simulink model "wsch_task"  (Simulink 3.00)
libraries: paramlib x357, logiclib x64, mathlib x53, execlib x22, genlib x3, analoglib x3

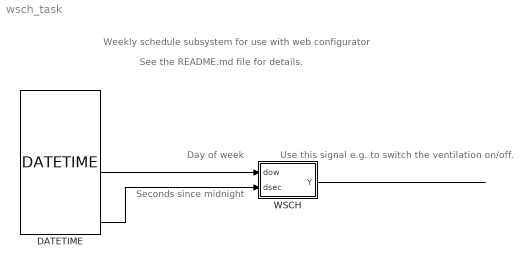
== system wsch_task ==
  note: Weekly schedule subsystem for use with web configurator
  note: See the README.md file for details.
  note: Day of week
  note: Seconds since midnight
  note: Use this signal e.g. to
      | switch the ventilation on/off.
  DATETIME : execlib/DATETIME  isetmode=1: OS clock  igetmode=1: OS clock  settol=1  setper=0  getper=1  FDOW=off  tz=1: Local time
  WSCH : Subsystem
      mask Type: REX sequence
  wires:
  DATETIME/8 -> WSCH/1(dow)
  DATETIME/13 -> WSCH/2(dsec)
  WSCH/1(Y) -> ?

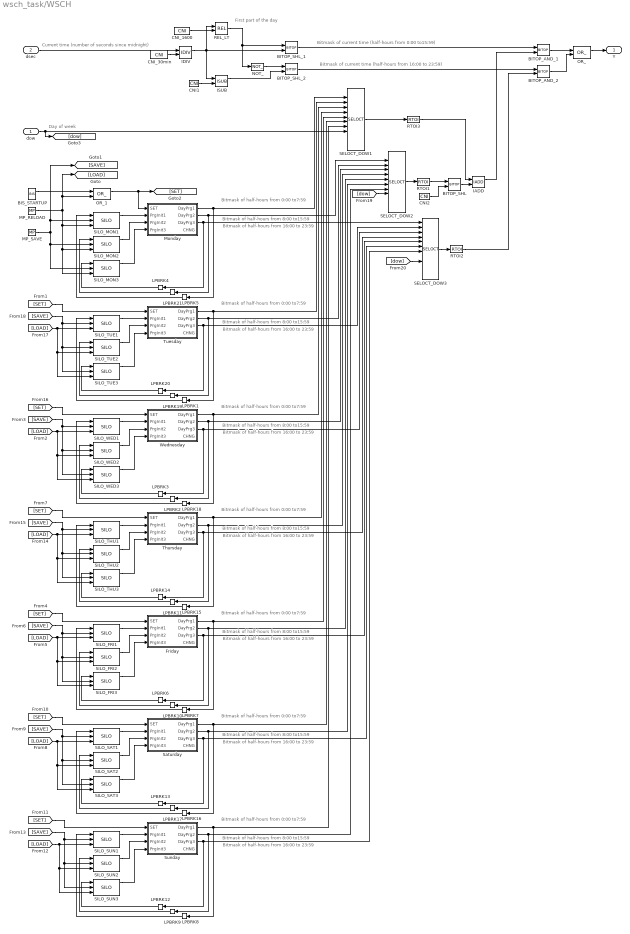
== system wsch_task/WSCH ==
  note: Bitmask of current time (half-hours from 0:00 to15:59)
  note: Bitmask of current time (half-hours from 16:00 to 23:59)
  note: First part of the day
  note: Bitmask of half-hours from 16:00 to 23:59
  note: Current time (number of seconds since midnight)
  note: Day of week
  note: Bitmask of half-hours from 0:00 to7:59
  note: Bitmask of half-hours from 8:00 to15:59
  note: Bitmask of half-hours from 16:00 to 23:59
  note: Bitmask of half-hours from 0:00 to7:59
  note: Bitmask of half-hours from 8:00 to15:59
  note: Bitmask of half-hours from 16:00 to 23:59
  note: Bitmask of half-hours from 0:00 to7:59
  note: Bitmask of half-hours from 8:00 to15:59
  note: Bitmask of half-hours from 16:00 to 23:59
  note: Bitmask of half-hours from 0:00 to7:59
  note: Bitmask of half-hours from 8:00 to15:59
  note: Bitmask of half-hours from 16:00 to 23:59
  note: Bitmask of half-hours from 0:00 to7:59
  note: Bitmask of half-hours from 8:00 to15:59
  note: Bitmask of half-hours from 16:00 to 23:59
  note: Bitmask of half-hours from 0:00 to7:59
  note: Bitmask of half-hours from 8:00 to15:59
  note: Bitmask of half-hours from 16:00 to 23:59
  note: Bitmask of half-hours from 0:00 to7:59
  note: Bitmask of half-hours from 8:00 to15:59
  dow : Inport  Port=1
  dsec : Inport  Port=2
  BIS_STARTUP : genlib/BIS  Y0=off  t1=1  t2=2  t3=0  t4=4  t5=5  t6=6  t7=7  t8=8  RPT=off
  BITOP_AND_1 : logiclib/BITOP  iop=3: Bit AND
  BITOP_AND_2 : logiclib/BITOP  iop=3: Bit AND
  BITOP_SHL : logiclib/BITOP  iop=5: Shift Left
  BITOP_SHL_1 : logiclib/BITOP  iop=5: Shift Left
  BITOP_SHL_2 : logiclib/BITOP  iop=5: Shift Left
  CNI1 : mathlib/CNI  icn=32
  CNI2 : mathlib/CNI  icn=16
  CNI_1600 : mathlib/CNI  icn=32
  CNI_30min : mathlib/CNI  icn=1800
  Friday : Subsystem
      mask Type: REX sequence
  IADD : mathlib/IADD  vtype=4: Long  SAT=off
  IDIV : mathlib/IDIV  vtype=4: Long  nerr=1
  ISUB : mathlib/ISUB  vtype=4: Long  SAT=off
  LPBRK{1..21} (21 alike) : execlib/LPBRK  Orientation=left
  MP_RELOAD : genlib/MP  pwidth=1  BSTATE=off  RPTF=off
  MP_SAVE : genlib/MP  pwidth=1  BSTATE=off  RPTF=off
  Monday : Subsystem
      mask Type: REX sequence
  NOT_ : logiclib/NOT_
  OR_ : logiclib/OR_
  OR_1 : logiclib/OR_
  REL_LT : mathlib/REL  irel=3: less than (<)
  RTOI1 : mathlib/RTOI
  RTOI2 : mathlib/RTOI
  RTOI3 : mathlib/RTOI
  SELOCT_DOW1 : analoglib/SELOCT  BINF=off
  SELOCT_DOW2 : analoglib/SELOCT  BINF=off
  SELOCT_DOW3 : analoglib/SELOCT  BINF=off
  SILO_FRI1 : paramlib/SILO  fname=wschfilt_fri1.dat  CSF=off  CLF=off  yerr=0
  SILO_FRI2 : paramlib/SILO  fname=wschfilt_fri2.dat  CSF=off  CLF=off  yerr=0
  SILO_FRI3 : paramlib/SILO  fname=wschfilt_fri3.dat  CSF=off  CLF=off  yerr=0
  SILO_MON1 : paramlib/SILO  fname=wschfilt_mon1.dat  CSF=off  CLF=off  yerr=0
  SILO_MON2 : paramlib/SILO  fname=wschfilt_mon2.dat  CSF=off  CLF=off  yerr=0
  SILO_MON3 : paramlib/SILO  fname=wschfilt_mon3.dat  CSF=off  CLF=off  yerr=0
  SILO_SAT1 : paramlib/SILO  fname=wschfilt_sat1.dat  CSF=off  CLF=off  yerr=0
  SILO_SAT2 : paramlib/SILO  fname=wschfilt_sat2.dat  CSF=off  CLF=off  yerr=0
  SILO_SAT3 : paramlib/SILO  fname=wschfilt_sat3.dat  CSF=off  CLF=off  yerr=0
  SILO_SUN1 : paramlib/SILO  fname=wschfilt_sun1.dat  CSF=off  CLF=off  yerr=0
  SILO_SUN2 : paramlib/SILO  fname=wschfilt_sun2.dat  CSF=off  CLF=off  yerr=0
  SILO_SUN3 : paramlib/SILO  fname=wschfilt_sun3.dat  CSF=off  CLF=off  yerr=0
  SILO_THU1 : paramlib/SILO  fname=wschfilt_thu1.dat  CSF=off  CLF=off  yerr=0
  SILO_THU2 : paramlib/SILO  fname=wschfilt_thu2.dat  CSF=off  CLF=off  yerr=0
  SILO_THU3 : paramlib/SILO  fname=wschfilt_thu3.dat  CSF=off  CLF=off  yerr=0
  SILO_TUE1 : paramlib/SILO  fname=wschfilt_tue1.dat  CSF=off  CLF=off  yerr=0
  SILO_TUE2 : paramlib/SILO  fname=wschfilt_tue2.dat  CSF=off  CLF=off  yerr=0
  SILO_TUE3 : paramlib/SILO  fname=wschfilt_tue3.dat  CSF=off  CLF=off  yerr=0
  SILO_WED1 : paramlib/SILO  fname=wschfilt_wed1.dat  CSF=off  CLF=off  yerr=0
  SILO_WED2 : paramlib/SILO  fname=wschfilt_wed2.dat  CSF=off  CLF=off  yerr=0
  SILO_WED3 : paramlib/SILO  fname=wschfilt_wed3.dat  CSF=off  CLF=off  yerr=0
  Saturday : Subsystem
      mask Type: REX sequence
  Sunday : Subsystem
      mask Type: REX sequence
  Thursday : Subsystem
      mask Type: REX sequence
  Tuesday : Subsystem
      mask Type: REX sequence
  Wednesday : Subsystem
      mask Type: REX sequence
  Y : Outport  Port=1
  wires:
  BIS_STARTUP/1 -> OR_1/1
  BITOP_AND_1/1 -> OR_/1
  BITOP_AND_2/1 -> OR_/2
  BITOP_SHL/1 -> IADD/2
  BITOP_SHL_1/1 -> BITOP_AND_1/1
  BITOP_SHL_2/1 -> BITOP_AND_2/1
  CNI1/1 -> ISUB/2
  CNI2/1 -> BITOP_SHL/2
  CNI_1600/1 -> REL_LT/2
  CNI_30min/1 -> IDIV/2
  Friday/1(DayPrg1) -> LPBRK7/1, SELOCT_DOW1/6
  Friday/2(DayPrg2) -> LPBRK10/1, SELOCT_DOW2/6
  Friday/3(DayPrg3) -> LPBRK6/1, SELOCT_DOW3/5
  [SET] -> Tuesday/1(SET)
  [SET] -> Saturday/1(SET)
  [SET] -> Sunday/1(SET)
  [LOAD] -> SILO_SUN1/3, SILO_SUN2/3, SILO_SUN3/3
  [SAVE] -> SILO_SUN1/2, SILO_SUN2/2, SILO_SUN3/2
  [LOAD] -> SILO_THU1/3, SILO_THU2/3, SILO_THU3/3
  [SAVE] -> SILO_THU1/2, SILO_THU2/2, SILO_THU3/2
  [SET] -> Wednesday/1(SET)
  [LOAD] -> SILO_TUE1/3, SILO_TUE2/3, SILO_TUE3/3
  [SAVE] -> SILO_TUE1/2, SILO_TUE2/2, SILO_TUE3/2
  [dow] -> SELOCT_DOW2/9
  [LOAD] -> SILO_WED1/3, SILO_WED2/3, SILO_WED3/3
  [dow] -> SELOCT_DOW3/9
  [SAVE] -> SILO_WED1/2, SILO_WED2/2, SILO_WED3/2
  [SET] -> Friday/1(SET)
  [LOAD] -> SILO_FRI1/3, SILO_FRI2/3, SILO_FRI3/3
  [SAVE] -> SILO_FRI1/2, SILO_FRI2/2, SILO_FRI3/2
  [SET] -> Thursday/1(SET)
  [LOAD] -> SILO_SAT1/3, SILO_SAT2/3, SILO_SAT3/3
  [SAVE] -> SILO_SAT1/2, SILO_SAT2/2, SILO_SAT3/2
  IADD/1 -> BITOP_AND_1/2
  IDIV/1 -> BITOP_SHL_1/2, ISUB/1, REL_LT/1
  ISUB/1 -> BITOP_SHL_2/2
  LPBRK1/1 -> SILO_TUE1/1
  LPBRK10/1 -> SILO_FRI2/1
  LPBRK11/1 -> SILO_THU2/1
  LPBRK12/1 -> SILO_SUN3/1
  LPBRK13/1 -> SILO_SAT3/1
  LPBRK14/1 -> SILO_THU3/1
  LPBRK15/1 -> SILO_THU1/1
  LPBRK16/1 -> SILO_SAT1/1
  LPBRK17/1 -> SILO_SAT2/1
  LPBRK18/1 -> SILO_WED1/1
  LPBRK19/1 -> SILO_TUE2/1
  LPBRK2/1 -> SILO_WED2/1
  LPBRK20/1 -> SILO_TUE3/1
  LPBRK21/1 -> SILO_MON2/1
  LPBRK3/1 -> SILO_WED3/1
  LPBRK4/1 -> SILO_MON3/1
  LPBRK5/1 -> SILO_MON1/1
  LPBRK6/1 -> SILO_FRI3/1
  LPBRK7/1 -> SILO_FRI1/1
  LPBRK8/1 -> SILO_SUN1/1
  LPBRK9/1 -> SILO_SUN2/1
  MP_RELOAD/1 -> SILO_MON1/3, SILO_MON2/3, SILO_MON3/3, [LOAD], OR_1/2
  MP_SAVE/1 -> [SAVE], SILO_MON1/2, SILO_MON2/2, SILO_MON3/2
  Monday/1(DayPrg1) -> LPBRK5/1, SELOCT_DOW1/2
  Monday/2(DayPrg2) -> LPBRK21/1, SELOCT_DOW2/2
  Monday/3(DayPrg3) -> LPBRK4/1, SELOCT_DOW3/1
  NOT_/1 -> BITOP_SHL_2/1
  OR_/1 -> Y/1
  OR_1/1 -> [SET], Monday/1(SET)
  REL_LT/1 -> BITOP_SHL_1/1, NOT_/1
  RTOI1/1 -> BITOP_SHL/1
  RTOI2/1 -> BITOP_AND_2/2
  RTOI3/1 -> IADD/1
  SELOCT_DOW1/1 -> RTOI3/1
  SELOCT_DOW2/1 -> RTOI1/1
  SELOCT_DOW3/1 -> RTOI2/1
  SILO_FRI1/1 -> Friday/2(PrgInit1)
  SILO_FRI2/1 -> Friday/3(PrgInit2)
  SILO_FRI3/1 -> Friday/4(PrgInit3)
  SILO_MON1/1 -> Monday/2(PrgInit1)
  SILO_MON2/1 -> Monday/3(PrgInit2)
  SILO_MON3/1 -> Monday/4(PrgInit3)
  SILO_SAT1/1 -> Saturday/2(PrgInit1)
  SILO_SAT2/1 -> Saturday/3(PrgInit2)
  SILO_SAT3/1 -> Saturday/4(PrgInit3)
  SILO_SUN1/1 -> Sunday/2(PrgInit1)
  SILO_SUN2/1 -> Sunday/3(PrgInit2)
  SILO_SUN3/1 -> Sunday/4(PrgInit3)
  SILO_THU1/1 -> Thursday/2(PrgInit1)
  SILO_THU2/1 -> Thursday/3(PrgInit2)
  SILO_THU3/1 -> Thursday/4(PrgInit3)
  SILO_TUE1/1 -> Tuesday/2(PrgInit1)
  SILO_TUE2/1 -> Tuesday/3(PrgInit2)
  SILO_TUE3/1 -> Tuesday/4(PrgInit3)
  SILO_WED1/1 -> Wednesday/2(PrgInit1)
  SILO_WED2/1 -> Wednesday/3(PrgInit2)
  SILO_WED3/1 -> Wednesday/4(PrgInit3)
  Saturday/1(DayPrg1) -> LPBRK16/1, SELOCT_DOW1/7
  Saturday/2(DayPrg2) -> LPBRK17/1, SELOCT_DOW2/7
  Saturday/3(DayPrg3) -> LPBRK13/1, SELOCT_DOW3/6
  Sunday/1(DayPrg1) -> LPBRK8/1, SELOCT_DOW1/8
  Sunday/2(DayPrg2) -> LPBRK9/1, SELOCT_DOW2/8
  Sunday/3(DayPrg3) -> LPBRK12/1, SELOCT_DOW3/7
  Thursday/1(DayPrg1) -> LPBRK15/1, SELOCT_DOW1/5
  Thursday/2(DayPrg2) -> LPBRK11/1, SELOCT_DOW2/5
  Thursday/3(DayPrg3) -> LPBRK14/1, SELOCT_DOW3/4
  Tuesday/1(DayPrg1) -> LPBRK1/1, SELOCT_DOW1/3
  Tuesday/2(DayPrg2) -> LPBRK19/1, SELOCT_DOW2/3
  Tuesday/3(DayPrg3) -> LPBRK20/1, SELOCT_DOW3/2
  Wednesday/1(DayPrg1) -> LPBRK18/1, SELOCT_DOW1/4
  Wednesday/2(DayPrg2) -> LPBRK2/1, SELOCT_DOW2/4
  Wednesday/3(DayPrg3) -> LPBRK3/1, SELOCT_DOW3/3
  dow/1 -> [dow], SELOCT_DOW1/9
  dsec/1 -> IDIV/1

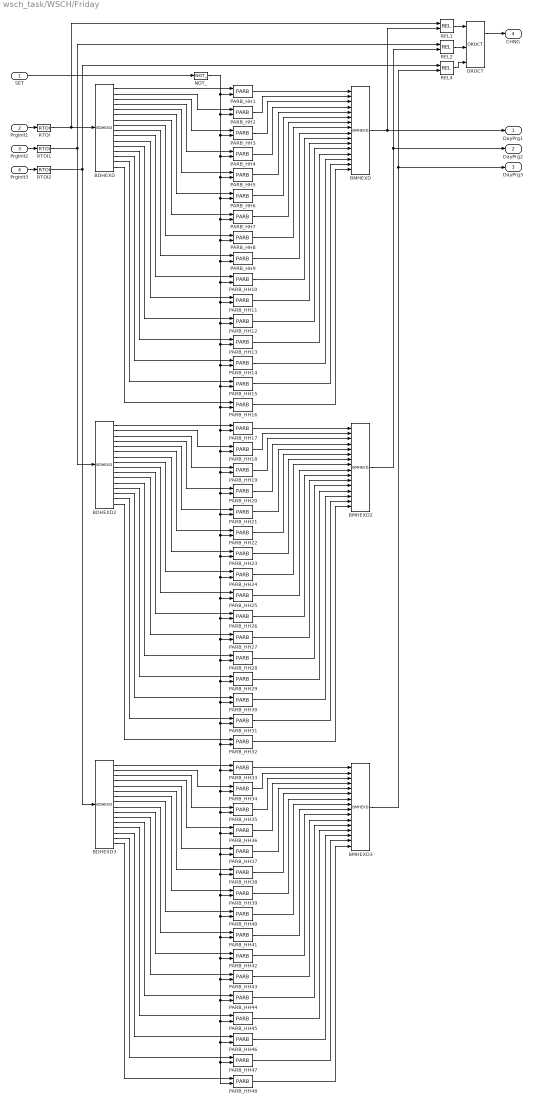
== system wsch_task/WSCH/Friday ==
  SET : Inport  Port=1
  PrgInit1 : Inport  Port=2
  PrgInit2 : Inport  Port=3
  PrgInit3 : Inport  Port=4
  BDHEXD : logiclib/BDHEXD  shift=0
  BDHEXD2 : logiclib/BDHEXD  shift=0
  BDHEXD3 : logiclib/BDHEXD  shift=0
  BMHEXD : logiclib/BMHEXD  shift=0
  BMHEXD2 : logiclib/BMHEXD  shift=0
  BMHEXD3 : logiclib/BMHEXD  shift=0
  NOT_ : logiclib/NOT_
  OROCT : logiclib/OROCT  nl=0
  PARB_HH{1..48} (48 alike) : paramlib/PARB  PAR=off
  REL1 : mathlib/REL  irel=2: inequality (!=)
  REL2 : mathlib/REL  irel=2: inequality (!=)
  REL4 : mathlib/REL  irel=2: inequality (!=)
  RTOI : mathlib/RTOI
  RTOI1 : mathlib/RTOI
  RTOI2 : mathlib/RTOI
  DayPrg1 : Outport  Port=1
  DayPrg2 : Outport  Port=2
  DayPrg3 : Outport  Port=3
  CHNG : Outport  Port=4
  wires:
  BDHEXD/1 -> PARB_HH1/1
  BDHEXD/2 -> PARB_HH2/1
  BDHEXD/3 -> PARB_HH3/1
  BDHEXD/4 -> PARB_HH4/1
  BDHEXD/5 -> PARB_HH5/1
  BDHEXD/6 -> PARB_HH6/1
  BDHEXD/7 -> PARB_HH7/1
  BDHEXD/8 -> PARB_HH8/1
  BDHEXD/9 -> PARB_HH9/1
  BDHEXD/10 -> PARB_HH10/1
  BDHEXD/11 -> PARB_HH11/1
  BDHEXD/12 -> PARB_HH12/1
  BDHEXD/13 -> PARB_HH13/1
  BDHEXD/14 -> PARB_HH14/1
  BDHEXD/15 -> PARB_HH15/1
  BDHEXD/16 -> PARB_HH16/1
  BDHEXD2/1 -> PARB_HH17/1
  BDHEXD2/2 -> PARB_HH18/1
  BDHEXD2/3 -> PARB_HH19/1
  BDHEXD2/4 -> PARB_HH20/1
  BDHEXD2/5 -> PARB_HH21/1
  BDHEXD2/6 -> PARB_HH22/1
  BDHEXD2/7 -> PARB_HH23/1
  BDHEXD2/8 -> PARB_HH24/1
  BDHEXD2/9 -> PARB_HH25/1
  BDHEXD2/10 -> PARB_HH26/1
  BDHEXD2/11 -> PARB_HH27/1
  BDHEXD2/12 -> PARB_HH28/1
  BDHEXD2/13 -> PARB_HH29/1
  BDHEXD2/14 -> PARB_HH30/1
  BDHEXD2/15 -> PARB_HH31/1
  BDHEXD2/16 -> PARB_HH32/1
  BDHEXD3/1 -> PARB_HH33/1
  BDHEXD3/2 -> PARB_HH34/1
  BDHEXD3/3 -> PARB_HH35/1
  BDHEXD3/4 -> PARB_HH36/1
  BDHEXD3/5 -> PARB_HH37/1
  BDHEXD3/6 -> PARB_HH38/1
  BDHEXD3/7 -> PARB_HH39/1
  BDHEXD3/8 -> PARB_HH40/1
  BDHEXD3/9 -> PARB_HH41/1
  BDHEXD3/10 -> PARB_HH42/1
  BDHEXD3/11 -> PARB_HH43/1
  BDHEXD3/12 -> PARB_HH44/1
  BDHEXD3/13 -> PARB_HH45/1
  BDHEXD3/14 -> PARB_HH46/1
  BDHEXD3/15 -> PARB_HH47/1
  BDHEXD3/16 -> PARB_HH48/1
  BMHEXD/1 -> DayPrg1/1, REL1/2
  BMHEXD2/1 -> DayPrg2/1, REL2/2
  BMHEXD3/1 -> DayPrg3/1, REL4/2
  NOT_/1 -> PARB_HH1/2, PARB_HH2/2, PARB_HH3/2, PARB_HH4/2, PARB_HH5/2, PARB_HH6/2, PARB_HH7/2, PARB_HH8/2, PARB_HH9/2, PARB_HH10/2, PARB_HH11/2, PARB_HH12/2, PARB_HH13/2, PARB_HH14/2, PARB_HH15/2, PARB_HH16/2, PARB_HH17/2, PARB_HH18/2, PARB_HH19/2, PARB_HH20/2, PARB_HH21/2, PARB_HH22/2, PARB_HH23/2, PARB_HH24/2, PARB_HH25/2, PARB_HH26/2, PARB_HH27/2, PARB_HH28/2, PARB_HH29/2, PARB_HH30/2, PARB_HH31/2, PARB_HH32/2, PARB_HH33/2, PARB_HH34/2, PARB_HH35/2, PARB_HH36/2, PARB_HH37/2, PARB_HH38/2, PARB_HH39/2, PARB_HH40/2, PARB_HH41/2, PARB_HH42/2, PARB_HH43/2, PARB_HH44/2, PARB_HH45/2, PARB_HH46/2, PARB_HH47/2, PARB_HH48/2
  OROCT/1 -> CHNG/1
  PARB_HH1/1 -> BMHEXD/1
  PARB_HH10/1 -> BMHEXD/10
  PARB_HH11/1 -> BMHEXD/11
  PARB_HH12/1 -> BMHEXD/12
  PARB_HH13/1 -> BMHEXD/13
  PARB_HH14/1 -> BMHEXD/14
  PARB_HH15/1 -> BMHEXD/15
  PARB_HH16/1 -> BMHEXD/16
  PARB_HH17/1 -> BMHEXD2/1
  PARB_HH18/1 -> BMHEXD2/2
  PARB_HH19/1 -> BMHEXD2/3
  PARB_HH2/1 -> BMHEXD/2
  PARB_HH20/1 -> BMHEXD2/4
  PARB_HH21/1 -> BMHEXD2/5
  PARB_HH22/1 -> BMHEXD2/6
  PARB_HH23/1 -> BMHEXD2/7
  PARB_HH24/1 -> BMHEXD2/8
  PARB_HH25/1 -> BMHEXD2/9
  PARB_HH26/1 -> BMHEXD2/10
  PARB_HH27/1 -> BMHEXD2/11
  PARB_HH28/1 -> BMHEXD2/12
  PARB_HH29/1 -> BMHEXD2/13
  PARB_HH3/1 -> BMHEXD/3
  PARB_HH30/1 -> BMHEXD2/14
  PARB_HH31/1 -> BMHEXD2/15
  PARB_HH32/1 -> BMHEXD2/16
  PARB_HH33/1 -> BMHEXD3/1
  PARB_HH34/1 -> BMHEXD3/2
  PARB_HH35/1 -> BMHEXD3/3
  PARB_HH36/1 -> BMHEXD3/4
  PARB_HH37/1 -> BMHEXD3/5
  PARB_HH38/1 -> BMHEXD3/6
  PARB_HH39/1 -> BMHEXD3/7
  PARB_HH4/1 -> BMHEXD/4
  PARB_HH40/1 -> BMHEXD3/8
  PARB_HH41/1 -> BMHEXD3/9
  PARB_HH42/1 -> BMHEXD3/10
  PARB_HH43/1 -> BMHEXD3/11
  PARB_HH44/1 -> BMHEXD3/12
  PARB_HH45/1 -> BMHEXD3/13
  PARB_HH46/1 -> BMHEXD3/14
  PARB_HH47/1 -> BMHEXD3/15
  PARB_HH48/1 -> BMHEXD3/16
  PARB_HH5/1 -> BMHEXD/5
  PARB_HH6/1 -> BMHEXD/6
  PARB_HH7/1 -> BMHEXD/7
  PARB_HH8/1 -> BMHEXD/8
  PARB_HH9/1 -> BMHEXD/9
  PrgInit1/1 -> RTOI/1
  PrgInit2/1 -> RTOI1/1
  PrgInit3/1 -> RTOI2/1
  REL1/1 -> OROCT/1
  REL2/1 -> OROCT/5
  REL4/1 -> OROCT/8
  RTOI/1 -> BDHEXD/1, REL1/1
  RTOI1/1 -> BDHEXD2/1, REL2/1
  RTOI2/1 -> BDHEXD3/1, REL4/1
  SET/1 -> NOT_/1

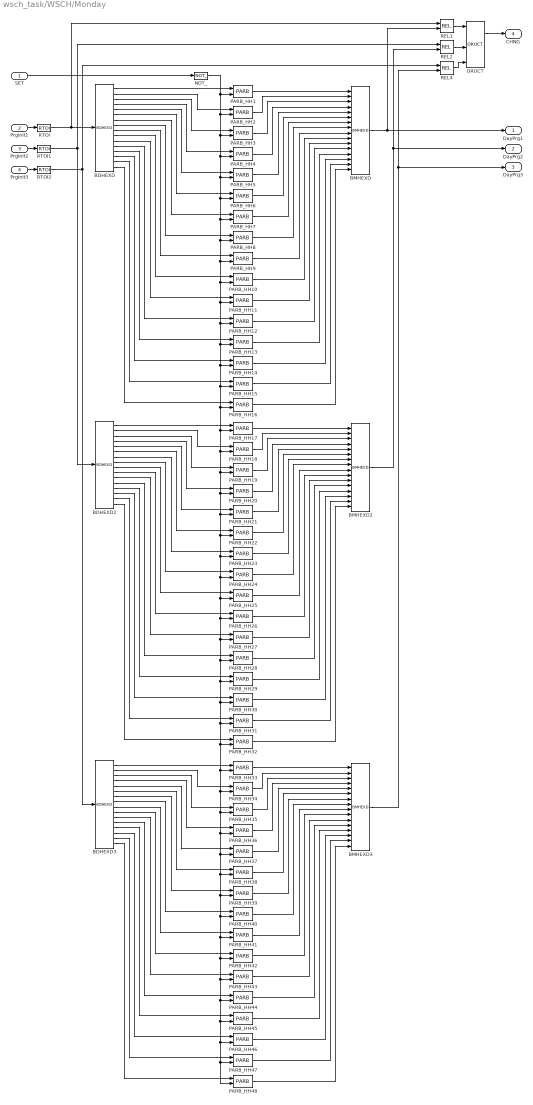
== system wsch_task/WSCH/Monday ==
  SET : Inport  Port=1
  PrgInit1 : Inport  Port=2
  PrgInit2 : Inport  Port=3
  PrgInit3 : Inport  Port=4
  BDHEXD : logiclib/BDHEXD  shift=0
  BDHEXD2 : logiclib/BDHEXD  shift=0
  BDHEXD3 : logiclib/BDHEXD  shift=0
  BMHEXD : logiclib/BMHEXD  shift=0
  BMHEXD2 : logiclib/BMHEXD  shift=0
  BMHEXD3 : logiclib/BMHEXD  shift=0
  NOT_ : logiclib/NOT_
  OROCT : logiclib/OROCT  nl=0
  PARB_HH{1..48} (48 alike) : paramlib/PARB  PAR=off
  REL1 : mathlib/REL  irel=2: inequality (!=)
  REL2 : mathlib/REL  irel=2: inequality (!=)
  REL4 : mathlib/REL  irel=2: inequality (!=)
  RTOI : mathlib/RTOI
  RTOI1 : mathlib/RTOI
  RTOI2 : mathlib/RTOI
  DayPrg1 : Outport  Port=1
  DayPrg2 : Outport  Port=2
  DayPrg3 : Outport  Port=3
  CHNG : Outport  Port=4
  wires:
  BDHEXD/1 -> PARB_HH1/1
  BDHEXD/2 -> PARB_HH2/1
  BDHEXD/3 -> PARB_HH3/1
  BDHEXD/4 -> PARB_HH4/1
  BDHEXD/5 -> PARB_HH5/1
  BDHEXD/6 -> PARB_HH6/1
  BDHEXD/7 -> PARB_HH7/1
  BDHEXD/8 -> PARB_HH8/1
  BDHEXD/9 -> PARB_HH9/1
  BDHEXD/10 -> PARB_HH10/1
  BDHEXD/11 -> PARB_HH11/1
  BDHEXD/12 -> PARB_HH12/1
  BDHEXD/13 -> PARB_HH13/1
  BDHEXD/14 -> PARB_HH14/1
  BDHEXD/15 -> PARB_HH15/1
  BDHEXD/16 -> PARB_HH16/1
  BDHEXD2/1 -> PARB_HH17/1
  BDHEXD2/2 -> PARB_HH18/1
  BDHEXD2/3 -> PARB_HH19/1
  BDHEXD2/4 -> PARB_HH20/1
  BDHEXD2/5 -> PARB_HH21/1
  BDHEXD2/6 -> PARB_HH22/1
  BDHEXD2/7 -> PARB_HH23/1
  BDHEXD2/8 -> PARB_HH24/1
  BDHEXD2/9 -> PARB_HH25/1
  BDHEXD2/10 -> PARB_HH26/1
  BDHEXD2/11 -> PARB_HH27/1
  BDHEXD2/12 -> PARB_HH28/1
  BDHEXD2/13 -> PARB_HH29/1
  BDHEXD2/14 -> PARB_HH30/1
  BDHEXD2/15 -> PARB_HH31/1
  BDHEXD2/16 -> PARB_HH32/1
  BDHEXD3/1 -> PARB_HH33/1
  BDHEXD3/2 -> PARB_HH34/1
  BDHEXD3/3 -> PARB_HH35/1
  BDHEXD3/4 -> PARB_HH36/1
  BDHEXD3/5 -> PARB_HH37/1
  BDHEXD3/6 -> PARB_HH38/1
  BDHEXD3/7 -> PARB_HH39/1
  BDHEXD3/8 -> PARB_HH40/1
  BDHEXD3/9 -> PARB_HH41/1
  BDHEXD3/10 -> PARB_HH42/1
  BDHEXD3/11 -> PARB_HH43/1
  BDHEXD3/12 -> PARB_HH44/1
  BDHEXD3/13 -> PARB_HH45/1
  BDHEXD3/14 -> PARB_HH46/1
  BDHEXD3/15 -> PARB_HH47/1
  BDHEXD3/16 -> PARB_HH48/1
  BMHEXD/1 -> DayPrg1/1, REL1/2
  BMHEXD2/1 -> DayPrg2/1, REL2/2
  BMHEXD3/1 -> DayPrg3/1, REL4/2
  NOT_/1 -> PARB_HH1/2, PARB_HH2/2, PARB_HH3/2, PARB_HH4/2, PARB_HH5/2, PARB_HH6/2, PARB_HH7/2, PARB_HH8/2, PARB_HH9/2, PARB_HH10/2, PARB_HH11/2, PARB_HH12/2, PARB_HH13/2, PARB_HH14/2, PARB_HH15/2, PARB_HH16/2, PARB_HH17/2, PARB_HH18/2, PARB_HH19/2, PARB_HH20/2, PARB_HH21/2, PARB_HH22/2, PARB_HH23/2, PARB_HH24/2, PARB_HH25/2, PARB_HH26/2, PARB_HH27/2, PARB_HH28/2, PARB_HH29/2, PARB_HH30/2, PARB_HH31/2, PARB_HH32/2, PARB_HH33/2, PARB_HH34/2, PARB_HH35/2, PARB_HH36/2, PARB_HH37/2, PARB_HH38/2, PARB_HH39/2, PARB_HH40/2, PARB_HH41/2, PARB_HH42/2, PARB_HH43/2, PARB_HH44/2, PARB_HH45/2, PARB_HH46/2, PARB_HH47/2, PARB_HH48/2
  OROCT/1 -> CHNG/1
  PARB_HH1/1 -> BMHEXD/1
  PARB_HH10/1 -> BMHEXD/10
  PARB_HH11/1 -> BMHEXD/11
  PARB_HH12/1 -> BMHEXD/12
  PARB_HH13/1 -> BMHEXD/13
  PARB_HH14/1 -> BMHEXD/14
  PARB_HH15/1 -> BMHEXD/15
  PARB_HH16/1 -> BMHEXD/16
  PARB_HH17/1 -> BMHEXD2/1
  PARB_HH18/1 -> BMHEXD2/2
  PARB_HH19/1 -> BMHEXD2/3
  PARB_HH2/1 -> BMHEXD/2
  PARB_HH20/1 -> BMHEXD2/4
  PARB_HH21/1 -> BMHEXD2/5
  PARB_HH22/1 -> BMHEXD2/6
  PARB_HH23/1 -> BMHEXD2/7
  PARB_HH24/1 -> BMHEXD2/8
  PARB_HH25/1 -> BMHEXD2/9
  PARB_HH26/1 -> BMHEXD2/10
  PARB_HH27/1 -> BMHEXD2/11
  PARB_HH28/1 -> BMHEXD2/12
  PARB_HH29/1 -> BMHEXD2/13
  PARB_HH3/1 -> BMHEXD/3
  PARB_HH30/1 -> BMHEXD2/14
  PARB_HH31/1 -> BMHEXD2/15
  PARB_HH32/1 -> BMHEXD2/16
  PARB_HH33/1 -> BMHEXD3/1
  PARB_HH34/1 -> BMHEXD3/2
  PARB_HH35/1 -> BMHEXD3/3
  PARB_HH36/1 -> BMHEXD3/4
  PARB_HH37/1 -> BMHEXD3/5
  PARB_HH38/1 -> BMHEXD3/6
  PARB_HH39/1 -> BMHEXD3/7
  PARB_HH4/1 -> BMHEXD/4
  PARB_HH40/1 -> BMHEXD3/8
  PARB_HH41/1 -> BMHEXD3/9
  PARB_HH42/1 -> BMHEXD3/10
  PARB_HH43/1 -> BMHEXD3/11
  PARB_HH44/1 -> BMHEXD3/12
  PARB_HH45/1 -> BMHEXD3/13
  PARB_HH46/1 -> BMHEXD3/14
  PARB_HH47/1 -> BMHEXD3/15
  PARB_HH48/1 -> BMHEXD3/16
  PARB_HH5/1 -> BMHEXD/5
  PARB_HH6/1 -> BMHEXD/6
  PARB_HH7/1 -> BMHEXD/7
  PARB_HH8/1 -> BMHEXD/8
  PARB_HH9/1 -> BMHEXD/9
  PrgInit1/1 -> RTOI/1
  PrgInit2/1 -> RTOI1/1
  PrgInit3/1 -> RTOI2/1
  REL1/1 -> OROCT/1
  REL2/1 -> OROCT/5
  REL4/1 -> OROCT/8
  RTOI/1 -> BDHEXD/1, REL1/1
  RTOI1/1 -> BDHEXD2/1, REL2/1
  RTOI2/1 -> BDHEXD3/1, REL4/1
  SET/1 -> NOT_/1

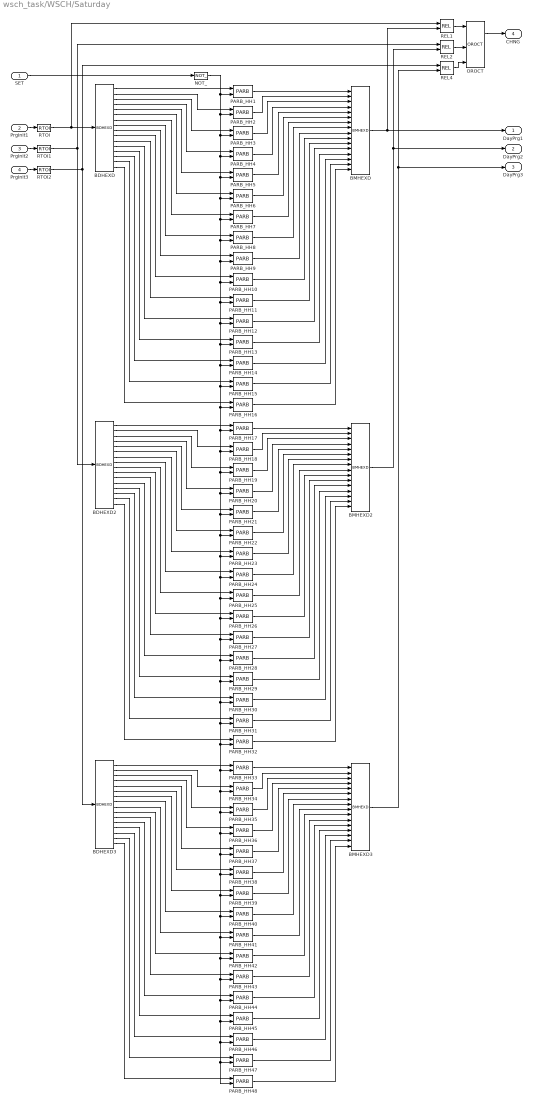
== system wsch_task/WSCH/Saturday ==
  SET : Inport  Port=1
  PrgInit1 : Inport  Port=2
  PrgInit2 : Inport  Port=3
  PrgInit3 : Inport  Port=4
  BDHEXD : logiclib/BDHEXD  shift=0
  BDHEXD2 : logiclib/BDHEXD  shift=0
  BDHEXD3 : logiclib/BDHEXD  shift=0
  BMHEXD : logiclib/BMHEXD  shift=0
  BMHEXD2 : logiclib/BMHEXD  shift=0
  BMHEXD3 : logiclib/BMHEXD  shift=0
  NOT_ : logiclib/NOT_
  OROCT : logiclib/OROCT  nl=0
  PARB_HH{1..48} (48 alike) : paramlib/PARB  PAR=off
  REL1 : mathlib/REL  irel=2: inequality (!=)
  REL2 : mathlib/REL  irel=2: inequality (!=)
  REL4 : mathlib/REL  irel=2: inequality (!=)
  RTOI : mathlib/RTOI
  RTOI1 : mathlib/RTOI
  RTOI2 : mathlib/RTOI
  DayPrg1 : Outport  Port=1
  DayPrg2 : Outport  Port=2
  DayPrg3 : Outport  Port=3
  CHNG : Outport  Port=4
  wires:
  BDHEXD/1 -> PARB_HH1/1
  BDHEXD/2 -> PARB_HH2/1
  BDHEXD/3 -> PARB_HH3/1
  BDHEXD/4 -> PARB_HH4/1
  BDHEXD/5 -> PARB_HH5/1
  BDHEXD/6 -> PARB_HH6/1
  BDHEXD/7 -> PARB_HH7/1
  BDHEXD/8 -> PARB_HH8/1
  BDHEXD/9 -> PARB_HH9/1
  BDHEXD/10 -> PARB_HH10/1
  BDHEXD/11 -> PARB_HH11/1
  BDHEXD/12 -> PARB_HH12/1
  BDHEXD/13 -> PARB_HH13/1
  BDHEXD/14 -> PARB_HH14/1
  BDHEXD/15 -> PARB_HH15/1
  BDHEXD/16 -> PARB_HH16/1
  BDHEXD2/1 -> PARB_HH17/1
  BDHEXD2/2 -> PARB_HH18/1
  BDHEXD2/3 -> PARB_HH19/1
  BDHEXD2/4 -> PARB_HH20/1
  BDHEXD2/5 -> PARB_HH21/1
  BDHEXD2/6 -> PARB_HH22/1
  BDHEXD2/7 -> PARB_HH23/1
  BDHEXD2/8 -> PARB_HH24/1
  BDHEXD2/9 -> PARB_HH25/1
  BDHEXD2/10 -> PARB_HH26/1
  BDHEXD2/11 -> PARB_HH27/1
  BDHEXD2/12 -> PARB_HH28/1
  BDHEXD2/13 -> PARB_HH29/1
  BDHEXD2/14 -> PARB_HH30/1
  BDHEXD2/15 -> PARB_HH31/1
  BDHEXD2/16 -> PARB_HH32/1
  BDHEXD3/1 -> PARB_HH33/1
  BDHEXD3/2 -> PARB_HH34/1
  BDHEXD3/3 -> PARB_HH35/1
  BDHEXD3/4 -> PARB_HH36/1
  BDHEXD3/5 -> PARB_HH37/1
  BDHEXD3/6 -> PARB_HH38/1
  BDHEXD3/7 -> PARB_HH39/1
  BDHEXD3/8 -> PARB_HH40/1
  BDHEXD3/9 -> PARB_HH41/1
  BDHEXD3/10 -> PARB_HH42/1
  BDHEXD3/11 -> PARB_HH43/1
  BDHEXD3/12 -> PARB_HH44/1
  BDHEXD3/13 -> PARB_HH45/1
  BDHEXD3/14 -> PARB_HH46/1
  BDHEXD3/15 -> PARB_HH47/1
  BDHEXD3/16 -> PARB_HH48/1
  BMHEXD/1 -> DayPrg1/1, REL1/2
  BMHEXD2/1 -> DayPrg2/1, REL2/2
  BMHEXD3/1 -> DayPrg3/1, REL4/2
  NOT_/1 -> PARB_HH1/2, PARB_HH2/2, PARB_HH3/2, PARB_HH4/2, PARB_HH5/2, PARB_HH6/2, PARB_HH7/2, PARB_HH8/2, PARB_HH9/2, PARB_HH10/2, PARB_HH11/2, PARB_HH12/2, PARB_HH13/2, PARB_HH14/2, PARB_HH15/2, PARB_HH16/2, PARB_HH17/2, PARB_HH18/2, PARB_HH19/2, PARB_HH20/2, PARB_HH21/2, PARB_HH22/2, PARB_HH23/2, PARB_HH24/2, PARB_HH25/2, PARB_HH26/2, PARB_HH27/2, PARB_HH28/2, PARB_HH29/2, PARB_HH30/2, PARB_HH31/2, PARB_HH32/2, PARB_HH33/2, PARB_HH34/2, PARB_HH35/2, PARB_HH36/2, PARB_HH37/2, PARB_HH38/2, PARB_HH39/2, PARB_HH40/2, PARB_HH41/2, PARB_HH42/2, PARB_HH43/2, PARB_HH44/2, PARB_HH45/2, PARB_HH46/2, PARB_HH47/2, PARB_HH48/2
  OROCT/1 -> CHNG/1
  PARB_HH1/1 -> BMHEXD/1
  PARB_HH10/1 -> BMHEXD/10
  PARB_HH11/1 -> BMHEXD/11
  PARB_HH12/1 -> BMHEXD/12
  PARB_HH13/1 -> BMHEXD/13
  PARB_HH14/1 -> BMHEXD/14
  PARB_HH15/1 -> BMHEXD/15
  PARB_HH16/1 -> BMHEXD/16
  PARB_HH17/1 -> BMHEXD2/1
  PARB_HH18/1 -> BMHEXD2/2
  PARB_HH19/1 -> BMHEXD2/3
  PARB_HH2/1 -> BMHEXD/2
  PARB_HH20/1 -> BMHEXD2/4
  PARB_HH21/1 -> BMHEXD2/5
  PARB_HH22/1 -> BMHEXD2/6
  PARB_HH23/1 -> BMHEXD2/7
  PARB_HH24/1 -> BMHEXD2/8
  PARB_HH25/1 -> BMHEXD2/9
  PARB_HH26/1 -> BMHEXD2/10
  PARB_HH27/1 -> BMHEXD2/11
  PARB_HH28/1 -> BMHEXD2/12
  PARB_HH29/1 -> BMHEXD2/13
  PARB_HH3/1 -> BMHEXD/3
  PARB_HH30/1 -> BMHEXD2/14
  PARB_HH31/1 -> BMHEXD2/15
  PARB_HH32/1 -> BMHEXD2/16
  PARB_HH33/1 -> BMHEXD3/1
  PARB_HH34/1 -> BMHEXD3/2
  PARB_HH35/1 -> BMHEXD3/3
  PARB_HH36/1 -> BMHEXD3/4
  PARB_HH37/1 -> BMHEXD3/5
  PARB_HH38/1 -> BMHEXD3/6
  PARB_HH39/1 -> BMHEXD3/7
  PARB_HH4/1 -> BMHEXD/4
  PARB_HH40/1 -> BMHEXD3/8
  PARB_HH41/1 -> BMHEXD3/9
  PARB_HH42/1 -> BMHEXD3/10
  PARB_HH43/1 -> BMHEXD3/11
  PARB_HH44/1 -> BMHEXD3/12
  PARB_HH45/1 -> BMHEXD3/13
  PARB_HH46/1 -> BMHEXD3/14
  PARB_HH47/1 -> BMHEXD3/15
  PARB_HH48/1 -> BMHEXD3/16
  PARB_HH5/1 -> BMHEXD/5
  PARB_HH6/1 -> BMHEXD/6
  PARB_HH7/1 -> BMHEXD/7
  PARB_HH8/1 -> BMHEXD/8
  PARB_HH9/1 -> BMHEXD/9
  PrgInit1/1 -> RTOI/1
  PrgInit2/1 -> RTOI1/1
  PrgInit3/1 -> RTOI2/1
  REL1/1 -> OROCT/1
  REL2/1 -> OROCT/5
  REL4/1 -> OROCT/8
  RTOI/1 -> BDHEXD/1, REL1/1
  RTOI1/1 -> BDHEXD2/1, REL2/1
  RTOI2/1 -> BDHEXD3/1, REL4/1
  SET/1 -> NOT_/1

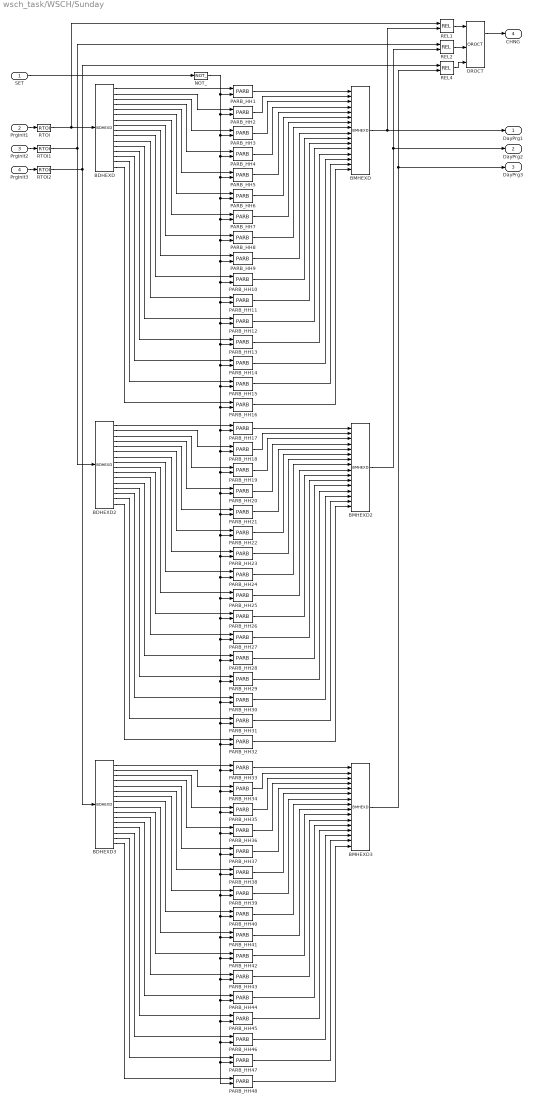
== system wsch_task/WSCH/Sunday ==
  SET : Inport  Port=1
  PrgInit1 : Inport  Port=2
  PrgInit2 : Inport  Port=3
  PrgInit3 : Inport  Port=4
  BDHEXD : logiclib/BDHEXD  shift=0
  BDHEXD2 : logiclib/BDHEXD  shift=0
  BDHEXD3 : logiclib/BDHEXD  shift=0
  BMHEXD : logiclib/BMHEXD  shift=0
  BMHEXD2 : logiclib/BMHEXD  shift=0
  BMHEXD3 : logiclib/BMHEXD  shift=0
  NOT_ : logiclib/NOT_
  OROCT : logiclib/OROCT  nl=0
  PARB_HH{1..48} (48 alike) : paramlib/PARB  PAR=off
  REL1 : mathlib/REL  irel=2: inequality (!=)
  REL2 : mathlib/REL  irel=2: inequality (!=)
  REL4 : mathlib/REL  irel=2: inequality (!=)
  RTOI : mathlib/RTOI
  RTOI1 : mathlib/RTOI
  RTOI2 : mathlib/RTOI
  DayPrg1 : Outport  Port=1
  DayPrg2 : Outport  Port=2
  DayPrg3 : Outport  Port=3
  CHNG : Outport  Port=4
  wires:
  BDHEXD/1 -> PARB_HH1/1
  BDHEXD/2 -> PARB_HH2/1
  BDHEXD/3 -> PARB_HH3/1
  BDHEXD/4 -> PARB_HH4/1
  BDHEXD/5 -> PARB_HH5/1
  BDHEXD/6 -> PARB_HH6/1
  BDHEXD/7 -> PARB_HH7/1
  BDHEXD/8 -> PARB_HH8/1
  BDHEXD/9 -> PARB_HH9/1
  BDHEXD/10 -> PARB_HH10/1
  BDHEXD/11 -> PARB_HH11/1
  BDHEXD/12 -> PARB_HH12/1
  BDHEXD/13 -> PARB_HH13/1
  BDHEXD/14 -> PARB_HH14/1
  BDHEXD/15 -> PARB_HH15/1
  BDHEXD/16 -> PARB_HH16/1
  BDHEXD2/1 -> PARB_HH17/1
  BDHEXD2/2 -> PARB_HH18/1
  BDHEXD2/3 -> PARB_HH19/1
  BDHEXD2/4 -> PARB_HH20/1
  BDHEXD2/5 -> PARB_HH21/1
  BDHEXD2/6 -> PARB_HH22/1
  BDHEXD2/7 -> PARB_HH23/1
  BDHEXD2/8 -> PARB_HH24/1
  BDHEXD2/9 -> PARB_HH25/1
  BDHEXD2/10 -> PARB_HH26/1
  BDHEXD2/11 -> PARB_HH27/1
  BDHEXD2/12 -> PARB_HH28/1
  BDHEXD2/13 -> PARB_HH29/1
  BDHEXD2/14 -> PARB_HH30/1
  BDHEXD2/15 -> PARB_HH31/1
  BDHEXD2/16 -> PARB_HH32/1
  BDHEXD3/1 -> PARB_HH33/1
  BDHEXD3/2 -> PARB_HH34/1
  BDHEXD3/3 -> PARB_HH35/1
  BDHEXD3/4 -> PARB_HH36/1
  BDHEXD3/5 -> PARB_HH37/1
  BDHEXD3/6 -> PARB_HH38/1
  BDHEXD3/7 -> PARB_HH39/1
  BDHEXD3/8 -> PARB_HH40/1
  BDHEXD3/9 -> PARB_HH41/1
  BDHEXD3/10 -> PARB_HH42/1
  BDHEXD3/11 -> PARB_HH43/1
  BDHEXD3/12 -> PARB_HH44/1
  BDHEXD3/13 -> PARB_HH45/1
  BDHEXD3/14 -> PARB_HH46/1
  BDHEXD3/15 -> PARB_HH47/1
  BDHEXD3/16 -> PARB_HH48/1
  BMHEXD/1 -> DayPrg1/1, REL1/2
  BMHEXD2/1 -> DayPrg2/1, REL2/2
  BMHEXD3/1 -> DayPrg3/1, REL4/2
  NOT_/1 -> PARB_HH1/2, PARB_HH2/2, PARB_HH3/2, PARB_HH4/2, PARB_HH5/2, PARB_HH6/2, PARB_HH7/2, PARB_HH8/2, PARB_HH9/2, PARB_HH10/2, PARB_HH11/2, PARB_HH12/2, PARB_HH13/2, PARB_HH14/2, PARB_HH15/2, PARB_HH16/2, PARB_HH17/2, PARB_HH18/2, PARB_HH19/2, PARB_HH20/2, PARB_HH21/2, PARB_HH22/2, PARB_HH23/2, PARB_HH24/2, PARB_HH25/2, PARB_HH26/2, PARB_HH27/2, PARB_HH28/2, PARB_HH29/2, PARB_HH30/2, PARB_HH31/2, PARB_HH32/2, PARB_HH33/2, PARB_HH34/2, PARB_HH35/2, PARB_HH36/2, PARB_HH37/2, PARB_HH38/2, PARB_HH39/2, PARB_HH40/2, PARB_HH41/2, PARB_HH42/2, PARB_HH43/2, PARB_HH44/2, PARB_HH45/2, PARB_HH46/2, PARB_HH47/2, PARB_HH48/2
  OROCT/1 -> CHNG/1
  PARB_HH1/1 -> BMHEXD/1
  PARB_HH10/1 -> BMHEXD/10
  PARB_HH11/1 -> BMHEXD/11
  PARB_HH12/1 -> BMHEXD/12
  PARB_HH13/1 -> BMHEXD/13
  PARB_HH14/1 -> BMHEXD/14
  PARB_HH15/1 -> BMHEXD/15
  PARB_HH16/1 -> BMHEXD/16
  PARB_HH17/1 -> BMHEXD2/1
  PARB_HH18/1 -> BMHEXD2/2
  PARB_HH19/1 -> BMHEXD2/3
  PARB_HH2/1 -> BMHEXD/2
  PARB_HH20/1 -> BMHEXD2/4
  PARB_HH21/1 -> BMHEXD2/5
  PARB_HH22/1 -> BMHEXD2/6
  PARB_HH23/1 -> BMHEXD2/7
  PARB_HH24/1 -> BMHEXD2/8
  PARB_HH25/1 -> BMHEXD2/9
  PARB_HH26/1 -> BMHEXD2/10
  PARB_HH27/1 -> BMHEXD2/11
  PARB_HH28/1 -> BMHEXD2/12
  PARB_HH29/1 -> BMHEXD2/13
  PARB_HH3/1 -> BMHEXD/3
  PARB_HH30/1 -> BMHEXD2/14
  PARB_HH31/1 -> BMHEXD2/15
  PARB_HH32/1 -> BMHEXD2/16
  PARB_HH33/1 -> BMHEXD3/1
  PARB_HH34/1 -> BMHEXD3/2
  PARB_HH35/1 -> BMHEXD3/3
  PARB_HH36/1 -> BMHEXD3/4
  PARB_HH37/1 -> BMHEXD3/5
  PARB_HH38/1 -> BMHEXD3/6
  PARB_HH39/1 -> BMHEXD3/7
  PARB_HH4/1 -> BMHEXD/4
  PARB_HH40/1 -> BMHEXD3/8
  PARB_HH41/1 -> BMHEXD3/9
  PARB_HH42/1 -> BMHEXD3/10
  PARB_HH43/1 -> BMHEXD3/11
  PARB_HH44/1 -> BMHEXD3/12
  PARB_HH45/1 -> BMHEXD3/13
  PARB_HH46/1 -> BMHEXD3/14
  PARB_HH47/1 -> BMHEXD3/15
  PARB_HH48/1 -> BMHEXD3/16
  PARB_HH5/1 -> BMHEXD/5
  PARB_HH6/1 -> BMHEXD/6
  PARB_HH7/1 -> BMHEXD/7
  PARB_HH8/1 -> BMHEXD/8
  PARB_HH9/1 -> BMHEXD/9
  PrgInit1/1 -> RTOI/1
  PrgInit2/1 -> RTOI1/1
  PrgInit3/1 -> RTOI2/1
  REL1/1 -> OROCT/1
  REL2/1 -> OROCT/5
  REL4/1 -> OROCT/8
  RTOI/1 -> BDHEXD/1, REL1/1
  RTOI1/1 -> BDHEXD2/1, REL2/1
  RTOI2/1 -> BDHEXD3/1, REL4/1
  SET/1 -> NOT_/1

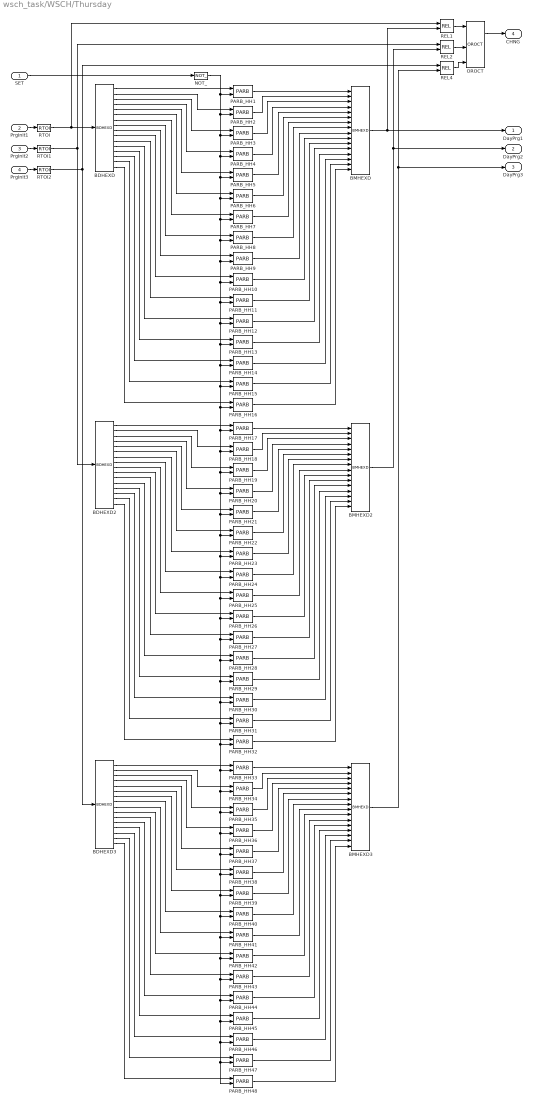
== system wsch_task/WSCH/Thursday ==
  SET : Inport  Port=1
  PrgInit1 : Inport  Port=2
  PrgInit2 : Inport  Port=3
  PrgInit3 : Inport  Port=4
  BDHEXD : logiclib/BDHEXD  shift=0
  BDHEXD2 : logiclib/BDHEXD  shift=0
  BDHEXD3 : logiclib/BDHEXD  shift=0
  BMHEXD : logiclib/BMHEXD  shift=0
  BMHEXD2 : logiclib/BMHEXD  shift=0
  BMHEXD3 : logiclib/BMHEXD  shift=0
  NOT_ : logiclib/NOT_
  OROCT : logiclib/OROCT  nl=0
  PARB_HH{1..48} (48 alike) : paramlib/PARB  PAR=off
  REL1 : mathlib/REL  irel=2: inequality (!=)
  REL2 : mathlib/REL  irel=2: inequality (!=)
  REL4 : mathlib/REL  irel=2: inequality (!=)
  RTOI : mathlib/RTOI
  RTOI1 : mathlib/RTOI
  RTOI2 : mathlib/RTOI
  DayPrg1 : Outport  Port=1
  DayPrg2 : Outport  Port=2
  DayPrg3 : Outport  Port=3
  CHNG : Outport  Port=4
  wires:
  BDHEXD/1 -> PARB_HH1/1
  BDHEXD/2 -> PARB_HH2/1
  BDHEXD/3 -> PARB_HH3/1
  BDHEXD/4 -> PARB_HH4/1
  BDHEXD/5 -> PARB_HH5/1
  BDHEXD/6 -> PARB_HH6/1
  BDHEXD/7 -> PARB_HH7/1
  BDHEXD/8 -> PARB_HH8/1
  BDHEXD/9 -> PARB_HH9/1
  BDHEXD/10 -> PARB_HH10/1
  BDHEXD/11 -> PARB_HH11/1
  BDHEXD/12 -> PARB_HH12/1
  BDHEXD/13 -> PARB_HH13/1
  BDHEXD/14 -> PARB_HH14/1
  BDHEXD/15 -> PARB_HH15/1
  BDHEXD/16 -> PARB_HH16/1
  BDHEXD2/1 -> PARB_HH17/1
  BDHEXD2/2 -> PARB_HH18/1
  BDHEXD2/3 -> PARB_HH19/1
  BDHEXD2/4 -> PARB_HH20/1
  BDHEXD2/5 -> PARB_HH21/1
  BDHEXD2/6 -> PARB_HH22/1
  BDHEXD2/7 -> PARB_HH23/1
  BDHEXD2/8 -> PARB_HH24/1
  BDHEXD2/9 -> PARB_HH25/1
  BDHEXD2/10 -> PARB_HH26/1
  BDHEXD2/11 -> PARB_HH27/1
  BDHEXD2/12 -> PARB_HH28/1
  BDHEXD2/13 -> PARB_HH29/1
  BDHEXD2/14 -> PARB_HH30/1
  BDHEXD2/15 -> PARB_HH31/1
  BDHEXD2/16 -> PARB_HH32/1
  BDHEXD3/1 -> PARB_HH33/1
  BDHEXD3/2 -> PARB_HH34/1
  BDHEXD3/3 -> PARB_HH35/1
  BDHEXD3/4 -> PARB_HH36/1
  BDHEXD3/5 -> PARB_HH37/1
  BDHEXD3/6 -> PARB_HH38/1
  BDHEXD3/7 -> PARB_HH39/1
  BDHEXD3/8 -> PARB_HH40/1
  BDHEXD3/9 -> PARB_HH41/1
  BDHEXD3/10 -> PARB_HH42/1
  BDHEXD3/11 -> PARB_HH43/1
  BDHEXD3/12 -> PARB_HH44/1
  BDHEXD3/13 -> PARB_HH45/1
  BDHEXD3/14 -> PARB_HH46/1
  BDHEXD3/15 -> PARB_HH47/1
  BDHEXD3/16 -> PARB_HH48/1
  BMHEXD/1 -> DayPrg1/1, REL1/2
  BMHEXD2/1 -> DayPrg2/1, REL2/2
  BMHEXD3/1 -> DayPrg3/1, REL4/2
  NOT_/1 -> PARB_HH1/2, PARB_HH2/2, PARB_HH3/2, PARB_HH4/2, PARB_HH5/2, PARB_HH6/2, PARB_HH7/2, PARB_HH8/2, PARB_HH9/2, PARB_HH10/2, PARB_HH11/2, PARB_HH12/2, PARB_HH13/2, PARB_HH14/2, PARB_HH15/2, PARB_HH16/2, PARB_HH17/2, PARB_HH18/2, PARB_HH19/2, PARB_HH20/2, PARB_HH21/2, PARB_HH22/2, PARB_HH23/2, PARB_HH24/2, PARB_HH25/2, PARB_HH26/2, PARB_HH27/2, PARB_HH28/2, PARB_HH29/2, PARB_HH30/2, PARB_HH31/2, PARB_HH32/2, PARB_HH33/2, PARB_HH34/2, PARB_HH35/2, PARB_HH36/2, PARB_HH37/2, PARB_HH38/2, PARB_HH39/2, PARB_HH40/2, PARB_HH41/2, PARB_HH42/2, PARB_HH43/2, PARB_HH44/2, PARB_HH45/2, PARB_HH46/2, PARB_HH47/2, PARB_HH48/2
  OROCT/1 -> CHNG/1
  PARB_HH1/1 -> BMHEXD/1
  PARB_HH10/1 -> BMHEXD/10
  PARB_HH11/1 -> BMHEXD/11
  PARB_HH12/1 -> BMHEXD/12
  PARB_HH13/1 -> BMHEXD/13
  PARB_HH14/1 -> BMHEXD/14
  PARB_HH15/1 -> BMHEXD/15
  PARB_HH16/1 -> BMHEXD/16
  PARB_HH17/1 -> BMHEXD2/1
  PARB_HH18/1 -> BMHEXD2/2
  PARB_HH19/1 -> BMHEXD2/3
  PARB_HH2/1 -> BMHEXD/2
  PARB_HH20/1 -> BMHEXD2/4
  PARB_HH21/1 -> BMHEXD2/5
  PARB_HH22/1 -> BMHEXD2/6
  PARB_HH23/1 -> BMHEXD2/7
  PARB_HH24/1 -> BMHEXD2/8
  PARB_HH25/1 -> BMHEXD2/9
  PARB_HH26/1 -> BMHEXD2/10
  PARB_HH27/1 -> BMHEXD2/11
  PARB_HH28/1 -> BMHEXD2/12
  PARB_HH29/1 -> BMHEXD2/13
  PARB_HH3/1 -> BMHEXD/3
  PARB_HH30/1 -> BMHEXD2/14
  PARB_HH31/1 -> BMHEXD2/15
  PARB_HH32/1 -> BMHEXD2/16
  PARB_HH33/1 -> BMHEXD3/1
  PARB_HH34/1 -> BMHEXD3/2
  PARB_HH35/1 -> BMHEXD3/3
  PARB_HH36/1 -> BMHEXD3/4
  PARB_HH37/1 -> BMHEXD3/5
  PARB_HH38/1 -> BMHEXD3/6
  PARB_HH39/1 -> BMHEXD3/7
  PARB_HH4/1 -> BMHEXD/4
  PARB_HH40/1 -> BMHEXD3/8
  PARB_HH41/1 -> BMHEXD3/9
  PARB_HH42/1 -> BMHEXD3/10
  PARB_HH43/1 -> BMHEXD3/11
  PARB_HH44/1 -> BMHEXD3/12
  PARB_HH45/1 -> BMHEXD3/13
  PARB_HH46/1 -> BMHEXD3/14
  PARB_HH47/1 -> BMHEXD3/15
  PARB_HH48/1 -> BMHEXD3/16
  PARB_HH5/1 -> BMHEXD/5
  PARB_HH6/1 -> BMHEXD/6
  PARB_HH7/1 -> BMHEXD/7
  PARB_HH8/1 -> BMHEXD/8
  PARB_HH9/1 -> BMHEXD/9
  PrgInit1/1 -> RTOI/1
  PrgInit2/1 -> RTOI1/1
  PrgInit3/1 -> RTOI2/1
  REL1/1 -> OROCT/1
  REL2/1 -> OROCT/5
  REL4/1 -> OROCT/8
  RTOI/1 -> BDHEXD/1, REL1/1
  RTOI1/1 -> BDHEXD2/1, REL2/1
  RTOI2/1 -> BDHEXD3/1, REL4/1
  SET/1 -> NOT_/1

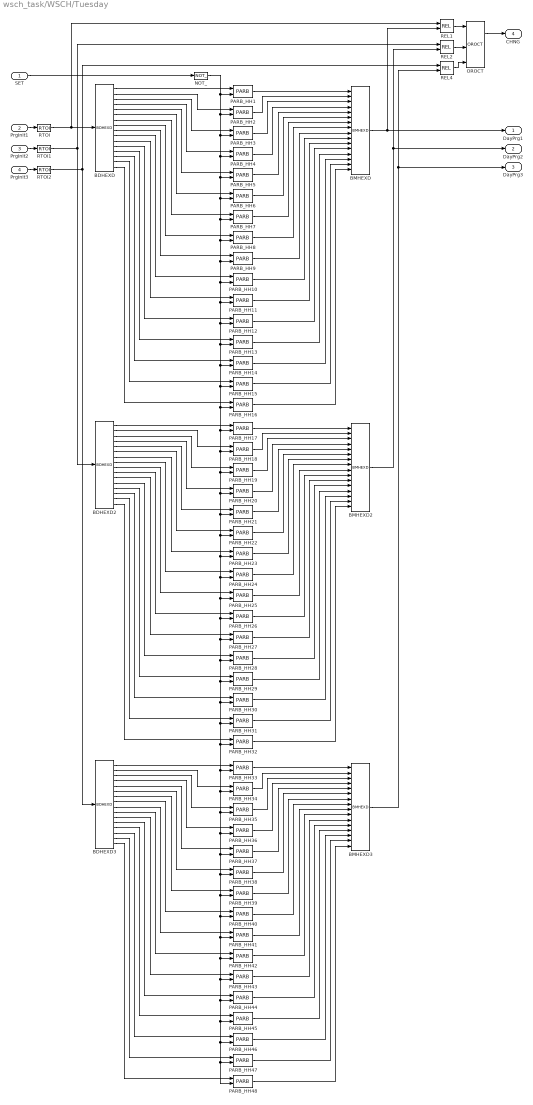
== system wsch_task/WSCH/Tuesday ==
  SET : Inport  Port=1
  PrgInit1 : Inport  Port=2
  PrgInit2 : Inport  Port=3
  PrgInit3 : Inport  Port=4
  BDHEXD : logiclib/BDHEXD  shift=0
  BDHEXD2 : logiclib/BDHEXD  shift=0
  BDHEXD3 : logiclib/BDHEXD  shift=0
  BMHEXD : logiclib/BMHEXD  shift=0
  BMHEXD2 : logiclib/BMHEXD  shift=0
  BMHEXD3 : logiclib/BMHEXD  shift=0
  NOT_ : logiclib/NOT_
  OROCT : logiclib/OROCT  nl=0
  PARB_HH{1..48} (48 alike) : paramlib/PARB  PAR=off
  REL1 : mathlib/REL  irel=2: inequality (!=)
  REL2 : mathlib/REL  irel=2: inequality (!=)
  REL4 : mathlib/REL  irel=2: inequality (!=)
  RTOI : mathlib/RTOI
  RTOI1 : mathlib/RTOI
  RTOI2 : mathlib/RTOI
  DayPrg1 : Outport  Port=1
  DayPrg2 : Outport  Port=2
  DayPrg3 : Outport  Port=3
  CHNG : Outport  Port=4
  wires:
  BDHEXD/1 -> PARB_HH1/1
  BDHEXD/2 -> PARB_HH2/1
  BDHEXD/3 -> PARB_HH3/1
  BDHEXD/4 -> PARB_HH4/1
  BDHEXD/5 -> PARB_HH5/1
  BDHEXD/6 -> PARB_HH6/1
  BDHEXD/7 -> PARB_HH7/1
  BDHEXD/8 -> PARB_HH8/1
  BDHEXD/9 -> PARB_HH9/1
  BDHEXD/10 -> PARB_HH10/1
  BDHEXD/11 -> PARB_HH11/1
  BDHEXD/12 -> PARB_HH12/1
  BDHEXD/13 -> PARB_HH13/1
  BDHEXD/14 -> PARB_HH14/1
  BDHEXD/15 -> PARB_HH15/1
  BDHEXD/16 -> PARB_HH16/1
  BDHEXD2/1 -> PARB_HH17/1
  BDHEXD2/2 -> PARB_HH18/1
  BDHEXD2/3 -> PARB_HH19/1
  BDHEXD2/4 -> PARB_HH20/1
  BDHEXD2/5 -> PARB_HH21/1
  BDHEXD2/6 -> PARB_HH22/1
  BDHEXD2/7 -> PARB_HH23/1
  BDHEXD2/8 -> PARB_HH24/1
  BDHEXD2/9 -> PARB_HH25/1
  BDHEXD2/10 -> PARB_HH26/1
  BDHEXD2/11 -> PARB_HH27/1
  BDHEXD2/12 -> PARB_HH28/1
  BDHEXD2/13 -> PARB_HH29/1
  BDHEXD2/14 -> PARB_HH30/1
  BDHEXD2/15 -> PARB_HH31/1
  BDHEXD2/16 -> PARB_HH32/1
  BDHEXD3/1 -> PARB_HH33/1
  BDHEXD3/2 -> PARB_HH34/1
  BDHEXD3/3 -> PARB_HH35/1
  BDHEXD3/4 -> PARB_HH36/1
  BDHEXD3/5 -> PARB_HH37/1
  BDHEXD3/6 -> PARB_HH38/1
  BDHEXD3/7 -> PARB_HH39/1
  BDHEXD3/8 -> PARB_HH40/1
  BDHEXD3/9 -> PARB_HH41/1
  BDHEXD3/10 -> PARB_HH42/1
  BDHEXD3/11 -> PARB_HH43/1
  BDHEXD3/12 -> PARB_HH44/1
  BDHEXD3/13 -> PARB_HH45/1
  BDHEXD3/14 -> PARB_HH46/1
  BDHEXD3/15 -> PARB_HH47/1
  BDHEXD3/16 -> PARB_HH48/1
  BMHEXD/1 -> DayPrg1/1, REL1/2
  BMHEXD2/1 -> DayPrg2/1, REL2/2
  BMHEXD3/1 -> DayPrg3/1, REL4/2
  NOT_/1 -> PARB_HH1/2, PARB_HH2/2, PARB_HH3/2, PARB_HH4/2, PARB_HH5/2, PARB_HH6/2, PARB_HH7/2, PARB_HH8/2, PARB_HH9/2, PARB_HH10/2, PARB_HH11/2, PARB_HH12/2, PARB_HH13/2, PARB_HH14/2, PARB_HH15/2, PARB_HH16/2, PARB_HH17/2, PARB_HH18/2, PARB_HH19/2, PARB_HH20/2, PARB_HH21/2, PARB_HH22/2, PARB_HH23/2, PARB_HH24/2, PARB_HH25/2, PARB_HH26/2, PARB_HH27/2, PARB_HH28/2, PARB_HH29/2, PARB_HH30/2, PARB_HH31/2, PARB_HH32/2, PARB_HH33/2, PARB_HH34/2, PARB_HH35/2, PARB_HH36/2, PARB_HH37/2, PARB_HH38/2, PARB_HH39/2, PARB_HH40/2, PARB_HH41/2, PARB_HH42/2, PARB_HH43/2, PARB_HH44/2, PARB_HH45/2, PARB_HH46/2, PARB_HH47/2, PARB_HH48/2
  OROCT/1 -> CHNG/1
  PARB_HH1/1 -> BMHEXD/1
  PARB_HH10/1 -> BMHEXD/10
  PARB_HH11/1 -> BMHEXD/11
  PARB_HH12/1 -> BMHEXD/12
  PARB_HH13/1 -> BMHEXD/13
  PARB_HH14/1 -> BMHEXD/14
  PARB_HH15/1 -> BMHEXD/15
  PARB_HH16/1 -> BMHEXD/16
  PARB_HH17/1 -> BMHEXD2/1
  PARB_HH18/1 -> BMHEXD2/2
  PARB_HH19/1 -> BMHEXD2/3
  PARB_HH2/1 -> BMHEXD/2
  PARB_HH20/1 -> BMHEXD2/4
  PARB_HH21/1 -> BMHEXD2/5
  PARB_HH22/1 -> BMHEXD2/6
  PARB_HH23/1 -> BMHEXD2/7
  PARB_HH24/1 -> BMHEXD2/8
  PARB_HH25/1 -> BMHEXD2/9
  PARB_HH26/1 -> BMHEXD2/10
  PARB_HH27/1 -> BMHEXD2/11
  PARB_HH28/1 -> BMHEXD2/12
  PARB_HH29/1 -> BMHEXD2/13
  PARB_HH3/1 -> BMHEXD/3
  PARB_HH30/1 -> BMHEXD2/14
  PARB_HH31/1 -> BMHEXD2/15
  PARB_HH32/1 -> BMHEXD2/16
  PARB_HH33/1 -> BMHEXD3/1
  PARB_HH34/1 -> BMHEXD3/2
  PARB_HH35/1 -> BMHEXD3/3
  PARB_HH36/1 -> BMHEXD3/4
  PARB_HH37/1 -> BMHEXD3/5
  PARB_HH38/1 -> BMHEXD3/6
  PARB_HH39/1 -> BMHEXD3/7
  PARB_HH4/1 -> BMHEXD/4
  PARB_HH40/1 -> BMHEXD3/8
  PARB_HH41/1 -> BMHEXD3/9
  PARB_HH42/1 -> BMHEXD3/10
  PARB_HH43/1 -> BMHEXD3/11
  PARB_HH44/1 -> BMHEXD3/12
  PARB_HH45/1 -> BMHEXD3/13
  PARB_HH46/1 -> BMHEXD3/14
  PARB_HH47/1 -> BMHEXD3/15
  PARB_HH48/1 -> BMHEXD3/16
  PARB_HH5/1 -> BMHEXD/5
  PARB_HH6/1 -> BMHEXD/6
  PARB_HH7/1 -> BMHEXD/7
  PARB_HH8/1 -> BMHEXD/8
  PARB_HH9/1 -> BMHEXD/9
  PrgInit1/1 -> RTOI/1
  PrgInit2/1 -> RTOI1/1
  PrgInit3/1 -> RTOI2/1
  REL1/1 -> OROCT/1
  REL2/1 -> OROCT/5
  REL4/1 -> OROCT/8
  RTOI/1 -> BDHEXD/1, REL1/1
  RTOI1/1 -> BDHEXD2/1, REL2/1
  RTOI2/1 -> BDHEXD3/1, REL4/1
  SET/1 -> NOT_/1

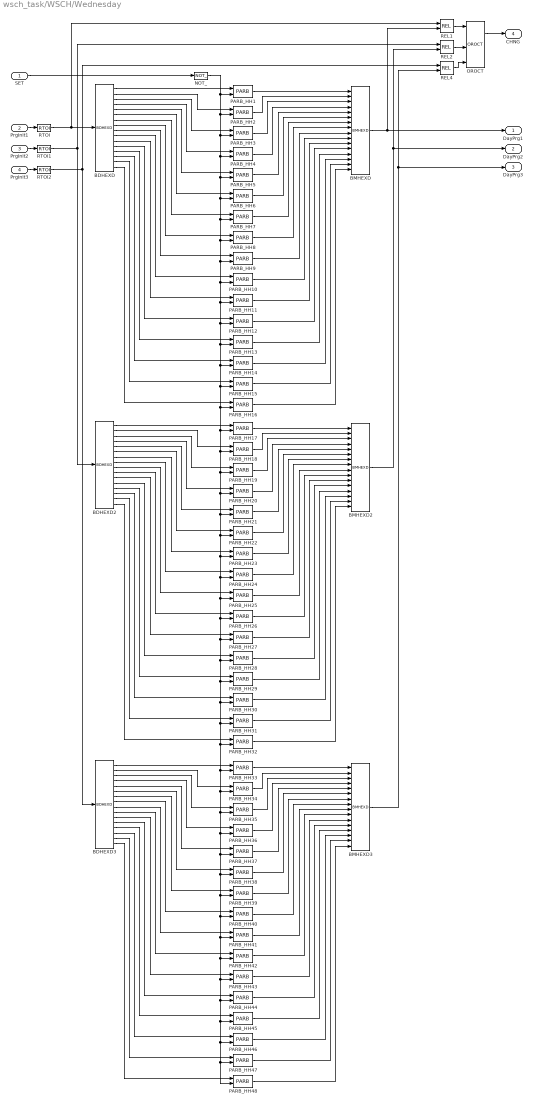
== system wsch_task/WSCH/Wednesday ==
  SET : Inport  Port=1
  PrgInit1 : Inport  Port=2
  PrgInit2 : Inport  Port=3
  PrgInit3 : Inport  Port=4
  BDHEXD : logiclib/BDHEXD  shift=0
  BDHEXD2 : logiclib/BDHEXD  shift=0
  BDHEXD3 : logiclib/BDHEXD  shift=0
  BMHEXD : logiclib/BMHEXD  shift=0
  BMHEXD2 : logiclib/BMHEXD  shift=0
  BMHEXD3 : logiclib/BMHEXD  shift=0
  NOT_ : logiclib/NOT_
  OROCT : logiclib/OROCT  nl=0
  PARB_HH{1..48} (48 alike) : paramlib/PARB  PAR=off
  REL1 : mathlib/REL  irel=2: inequality (!=)
  REL2 : mathlib/REL  irel=2: inequality (!=)
  REL4 : mathlib/REL  irel=2: inequality (!=)
  RTOI : mathlib/RTOI
  RTOI1 : mathlib/RTOI
  RTOI2 : mathlib/RTOI
  DayPrg1 : Outport  Port=1
  DayPrg2 : Outport  Port=2
  DayPrg3 : Outport  Port=3
  CHNG : Outport  Port=4
  wires:
  BDHEXD/1 -> PARB_HH1/1
  BDHEXD/2 -> PARB_HH2/1
  BDHEXD/3 -> PARB_HH3/1
  BDHEXD/4 -> PARB_HH4/1
  BDHEXD/5 -> PARB_HH5/1
  BDHEXD/6 -> PARB_HH6/1
  BDHEXD/7 -> PARB_HH7/1
  BDHEXD/8 -> PARB_HH8/1
  BDHEXD/9 -> PARB_HH9/1
  BDHEXD/10 -> PARB_HH10/1
  BDHEXD/11 -> PARB_HH11/1
  BDHEXD/12 -> PARB_HH12/1
  BDHEXD/13 -> PARB_HH13/1
  BDHEXD/14 -> PARB_HH14/1
  BDHEXD/15 -> PARB_HH15/1
  BDHEXD/16 -> PARB_HH16/1
  BDHEXD2/1 -> PARB_HH17/1
  BDHEXD2/2 -> PARB_HH18/1
  BDHEXD2/3 -> PARB_HH19/1
  BDHEXD2/4 -> PARB_HH20/1
  BDHEXD2/5 -> PARB_HH21/1
  BDHEXD2/6 -> PARB_HH22/1
  BDHEXD2/7 -> PARB_HH23/1
  BDHEXD2/8 -> PARB_HH24/1
  BDHEXD2/9 -> PARB_HH25/1
  BDHEXD2/10 -> PARB_HH26/1
  BDHEXD2/11 -> PARB_HH27/1
  BDHEXD2/12 -> PARB_HH28/1
  BDHEXD2/13 -> PARB_HH29/1
  BDHEXD2/14 -> PARB_HH30/1
  BDHEXD2/15 -> PARB_HH31/1
  BDHEXD2/16 -> PARB_HH32/1
  BDHEXD3/1 -> PARB_HH33/1
  BDHEXD3/2 -> PARB_HH34/1
  BDHEXD3/3 -> PARB_HH35/1
  BDHEXD3/4 -> PARB_HH36/1
  BDHEXD3/5 -> PARB_HH37/1
  BDHEXD3/6 -> PARB_HH38/1
  BDHEXD3/7 -> PARB_HH39/1
  BDHEXD3/8 -> PARB_HH40/1
  BDHEXD3/9 -> PARB_HH41/1
  BDHEXD3/10 -> PARB_HH42/1
  BDHEXD3/11 -> PARB_HH43/1
  BDHEXD3/12 -> PARB_HH44/1
  BDHEXD3/13 -> PARB_HH45/1
  BDHEXD3/14 -> PARB_HH46/1
  BDHEXD3/15 -> PARB_HH47/1
  BDHEXD3/16 -> PARB_HH48/1
  BMHEXD/1 -> DayPrg1/1, REL1/2
  BMHEXD2/1 -> DayPrg2/1, REL2/2
  BMHEXD3/1 -> DayPrg3/1, REL4/2
  NOT_/1 -> PARB_HH1/2, PARB_HH2/2, PARB_HH3/2, PARB_HH4/2, PARB_HH5/2, PARB_HH6/2, PARB_HH7/2, PARB_HH8/2, PARB_HH9/2, PARB_HH10/2, PARB_HH11/2, PARB_HH12/2, PARB_HH13/2, PARB_HH14/2, PARB_HH15/2, PARB_HH16/2, PARB_HH17/2, PARB_HH18/2, PARB_HH19/2, PARB_HH20/2, PARB_HH21/2, PARB_HH22/2, PARB_HH23/2, PARB_HH24/2, PARB_HH25/2, PARB_HH26/2, PARB_HH27/2, PARB_HH28/2, PARB_HH29/2, PARB_HH30/2, PARB_HH31/2, PARB_HH32/2, PARB_HH33/2, PARB_HH34/2, PARB_HH35/2, PARB_HH36/2, PARB_HH37/2, PARB_HH38/2, PARB_HH39/2, PARB_HH40/2, PARB_HH41/2, PARB_HH42/2, PARB_HH43/2, PARB_HH44/2, PARB_HH45/2, PARB_HH46/2, PARB_HH47/2, PARB_HH48/2
  OROCT/1 -> CHNG/1
  PARB_HH1/1 -> BMHEXD/1
  PARB_HH10/1 -> BMHEXD/10
  PARB_HH11/1 -> BMHEXD/11
  PARB_HH12/1 -> BMHEXD/12
  PARB_HH13/1 -> BMHEXD/13
  PARB_HH14/1 -> BMHEXD/14
  PARB_HH15/1 -> BMHEXD/15
  PARB_HH16/1 -> BMHEXD/16
  PARB_HH17/1 -> BMHEXD2/1
  PARB_HH18/1 -> BMHEXD2/2
  PARB_HH19/1 -> BMHEXD2/3
  PARB_HH2/1 -> BMHEXD/2
  PARB_HH20/1 -> BMHEXD2/4
  PARB_HH21/1 -> BMHEXD2/5
  PARB_HH22/1 -> BMHEXD2/6
  PARB_HH23/1 -> BMHEXD2/7
  PARB_HH24/1 -> BMHEXD2/8
  PARB_HH25/1 -> BMHEXD2/9
  PARB_HH26/1 -> BMHEXD2/10
  PARB_HH27/1 -> BMHEXD2/11
  PARB_HH28/1 -> BMHEXD2/12
  PARB_HH29/1 -> BMHEXD2/13
  PARB_HH3/1 -> BMHEXD/3
  PARB_HH30/1 -> BMHEXD2/14
  PARB_HH31/1 -> BMHEXD2/15
  PARB_HH32/1 -> BMHEXD2/16
  PARB_HH33/1 -> BMHEXD3/1
  PARB_HH34/1 -> BMHEXD3/2
  PARB_HH35/1 -> BMHEXD3/3
  PARB_HH36/1 -> BMHEXD3/4
  PARB_HH37/1 -> BMHEXD3/5
  PARB_HH38/1 -> BMHEXD3/6
  PARB_HH39/1 -> BMHEXD3/7
  PARB_HH4/1 -> BMHEXD/4
  PARB_HH40/1 -> BMHEXD3/8
  PARB_HH41/1 -> BMHEXD3/9
  PARB_HH42/1 -> BMHEXD3/10
  PARB_HH43/1 -> BMHEXD3/11
  PARB_HH44/1 -> BMHEXD3/12
  PARB_HH45/1 -> BMHEXD3/13
  PARB_HH46/1 -> BMHEXD3/14
  PARB_HH47/1 -> BMHEXD3/15
  PARB_HH48/1 -> BMHEXD3/16
  PARB_HH5/1 -> BMHEXD/5
  PARB_HH6/1 -> BMHEXD/6
  PARB_HH7/1 -> BMHEXD/7
  PARB_HH8/1 -> BMHEXD/8
  PARB_HH9/1 -> BMHEXD/9
  PrgInit1/1 -> RTOI/1
  PrgInit2/1 -> RTOI1/1
  PrgInit3/1 -> RTOI2/1
  REL1/1 -> OROCT/1
  REL2/1 -> OROCT/5
  REL4/1 -> OROCT/8
  RTOI/1 -> BDHEXD/1, REL1/1
  RTOI1/1 -> BDHEXD2/1, REL2/1
  RTOI2/1 -> BDHEXD3/1, REL4/1
  SET/1 -> NOT_/1
